simulink model "eovsa_corr_300mhz"  (R2012b)
settings: Solver=VariableStepDiscrete  SolverMode=SingleTasking  StartTime=0.0  StopTime=5000  RelTol=1e-3
undefined symbols (not defined in the file or in its folder): A, B, gcbh, PCIN, sfp, xlBlockLoadCallback, xlipgetpartsetting
libraries: xbsIndex_r4 x5996, casper_library_misc x52, simulink x33, dspsigops x24, xps_library x15, casper_library_delays x2
(part 3 of 65)

== system eovsa_corr_300mhz/FPGA_pps ==
  Slice29 : xbsIndex_r4/Slice  nbits=1  boolean_output=on  mode=Upper Bit Location + Width  bit1=0  base1=MSB of Input  bit0=0  base0=LSB of Input  dbl_ovrd=off  block_type=slice
  count_1sec : xbsIndex_r4/Counter  cnt_type=Count Limited  cnt_to=( fpga_clk * ( 10 ^ 6 ) ) - 1  operation=Up  start_count=0  cnt_by_val=1  arith_type=Unsigned  n_bits=ceil( log2( fpga_clk * ( 10 ^ 6 ) ) )  bin_pt=0  load_pin=off  rst=off  en=off  explicit_period=on  period=1  dbl_ovrd=off  use_behavioral_HDL=off  implementation=DSP48  block_type=counter
      settings: block_version=11.4
  edge_detect6 : Subsystem  AncestorBlock=casper_library_misc/edge_detect  mask(edge_detect){edge=Falling, polarity=Active High, x_in=[0 0.08 0.08 0.16 0.16 0.24 0.24 0.32 0.32 0.4], y_in=[1  1 -1 -1 -1 -1 -1 -1 -1 -1], x_out=[0.6 0.68 0.68 0.76 0.76 0.84 0.84 0.92 0.92 1], y_out=[-1 -1  1  1 -1 -1 -1 -1 -1 -1]}
      mask prompts: edge "Edge Type"; polarity "Output Polarity"; x_in "Input X Positions"; y_in "Input Y Positions"; x_out "Output X Positions"; y_out "Output Y Positions"
      mask help: Output is active for one-cycle after each edge of the specified type (i.e. rising, falling or both).
      mask init: same as eovsa_corr_300mhz/edge_detect1
      settings: AttributesFormatString=|
      | falling edges
      | active high
      mask Help: Output is active for one-cycle after each edge of the specified type (i.e. rising, falling, or both).  Latency is zero.
      mask TypeOptions edge: Rising | Falling | Both
      mask TypeOptions polarity: Active High | Active Low
      mask Display:
      | plot(x_in_num,0.5+y_in_num*0.2);
      | plot(x_out_num,0.5+y_out_num*0.2);
  pps : Outport
  wires:
  count_1sec/1 -> Slice29/1
  Slice29/1 -> edge_detect6/1(in)
  edge_detect6/1(out) -> pps/1

== system eovsa_corr_300mhz/Subsystem ==
  In1 : Inport
  Delay{16..23,28..30,32,34,37} (14 alike) : xbsIndex_r4/Delay  rst=off  infoeditControl=Selection of Reset will increase slice count due to use of real FFs and instead of SRLs  en=off  latency=1  dbl_ovrd=off  reg_retiming=off  block_type=delay
      settings: block_version=11.4
  Out1 : Outport
  Out2 : Outport  Port=2
  Out3 : Outport  Port=3
  Out4 : Outport  Port=4
  Out5 : Outport  Port=5
  Out6 : Outport  Port=6
  Out7 : Outport  Port=7
  Out8 : Outport  Port=8
  wires:
  Delay21/1 -> Delay37/1, Delay34/1
  Delay19/1 -> Delay28/1, Delay29/1
  Delay29/1 -> Out4/1
  Delay32/1 -> Out6/1
  Delay30/1 -> Out5/1
  In1/1 -> Delay16/1, Delay17/1
  Delay18/1 -> Delay22/1, Delay23/1
  Delay20/1 -> Delay32/1, Delay30/1
  Delay22/1 -> Out1/1
  Delay34/1 -> Out7/1
  Delay23/1 -> Out2/1
  Delay16/1 -> Delay19/1, Delay18/1
  Delay28/1 -> Out3/1
  Delay17/1 -> Delay21/1, Delay20/1
  Delay37/1 -> Out8/1

== system eovsa_corr_300mhz/acc_sync ==
  note: Count number of ADC overflows in an accumulation.
  sync : Inport
  acc_len : Inport  Port=2
  acc_start_skip : Inport  Port=3
  adc_over : Inport  Port=4
  AddSub : xbsIndex_r4/AddSub  mode=Addition  use_carryin=off  use_carryout=off  en=off  latency=1  precision=User Defined  arith_type=Unsigned  n_bits=16  bin_pt=0  quantization=Truncate  overflow=Wrap  dbl_ovrd=off  use_behavioral_HDL=off  hw_selection=DSP48  pipelined=off  block_type=addsub
  Count_FFT_frames1 : xbsIndex_r4/Counter  cnt_type=Free Running  cnt_to=0  operation=Up  start_count=0  cnt_by_val=1  arith_type=Unsigned  n_bits=32  bin_pt=0  load_pin=off  rst=on  en=on  explicit_period=off  period=1  dbl_ovrd=off  use_behavioral_HDL=off  implementation=DSP48  use_rpm=off  block_type=counter
  Delay{1,3..6,8..11} (9 alike) : xbsIndex_r4/Delay  rst=off  infoeditControl=Selection of Reset will increase slice count due to use of real FFs and instead of SRLs  en=off  latency=1  dbl_ovrd=off  reg_retiming=off  block_type=delay
      settings: block_version=11.4
  Delay2 : xbsIndex_r4/Delay  rst=off  infoeditControl=Selection of Reset will increase slice count due to use of real FFs and instead of SRLs  en=off  latency=2  dbl_ovrd=off  reg_retiming=on  block_type=delay
      settings: block_version=11.4
  Delay7 : xbsIndex_r4/Delay  rst=off  infoeditControl=Selection of Reset will increase slice count due to use of real FFs and instead of SRLs  en=off  latency=2  dbl_ovrd=off  reg_retiming=off  block_type=delay
      settings: block_version=11.4
  Register1 : xbsIndex_r4/Register  init=0  rst=off  en=on  dbl_ovrd=off  block_type=register
      settings: block_version=11.4
  Relational2 : xbsIndex_r4/Relational  mode=a=b  en=off  latency=1  dbl_ovrd=off  block_type=relational
  Relational3 : xbsIndex_r4/Relational  mode=a=b  en=off  latency=1  dbl_ovrd=off  block_type=relational
  adc_overflow_count : xbsIndex_r4/Counter  cnt_type=Free Running  cnt_to=5  operation=Up  start_count=0  cnt_by_val=1  arith_type=Unsigned  n_bits=32  bin_pt=0  load_pin=off  rst=on  en=on  explicit_period=off  period=1  dbl_ovrd=off  use_behavioral_HDL=off  implementation=DSP48  use_rpm=off  block_type=counter
  edge_detect : Subsystem  AncestorBlock=casper_library_misc/edge_detect  mask(edge_detect){edge=Rising, polarity=Active High, x_in=[0 0.08 0.08 0.16 0.16 0.24 0.24 0.32 0.32 0.4], y_in=[-1 -1  1  1  1  1  1  1  1  1], x_out=[0.6 0.68 0.68 0.76 0.76 0.84 0.84 0.92 0.92 1], y_out=[-1 -1  1  1 -1 -1 -1 -1 -1 -1]}
      mask prompts: edge "Edge Type"; polarity "Output Polarity"; x_in "Input X Positions"; y_in "Input Y Positions"; x_out "Output X Positions"; y_out "Output Y Positions"
      mask help: Output is active for one-cycle after each edge of the specified type (i.e. rising, falling or both).
      mask init: same as eovsa_corr_300mhz/edge_detect1
      settings: AttributesFormatString=|
      | rising edges
      | active high
      mask Help: Output is active for one-cycle after each edge of the specified type (i.e. rising, falling, or both).  Latency is zero.
      mask TypeOptions edge: Rising | Falling | Both
      mask TypeOptions polarity: Active High | Active Low
      mask Display:
      | plot(x_in_num,0.5+y_in_num*0.2);
      | plot(x_out_num,0.5+y_out_num*0.2);
  edge_detect1 : Subsystem  AncestorBlock=casper_library_misc/edge_detect  mask(edge_detect){edge=Rising, polarity=Active High, x_in=[0 0.08 0.08 0.16 0.16 0.24 0.24 0.32 0.32 0.4], y_in=[-1 -1  1  1  1  1  1  1  1  1], x_out=[0.6 0.68 0.68 0.76 0.76 0.84 0.84 0.92 0.92 1], y_out=[-1 -1  1  1 -1 -1 -1 -1 -1 -1]}
      mask prompts: edge "Edge Type"; polarity "Output Polarity"; x_in "Input X Positions"; y_in "Input Y Positions"; x_out "Output X Positions"; y_out "Output Y Positions"
      mask help: Output is active for one-cycle after each edge of the specified type (i.e. rising, falling or both).
      mask init: same as eovsa_corr_300mhz/edge_detect1
      settings: AttributesFormatString=|
      | rising edges
      | active high
      mask Help: Output is active for one-cycle after each edge of the specified type (i.e. rising, falling, or both).  Latency is zero.
      mask TypeOptions edge: Rising | Falling | Both
      mask TypeOptions polarity: Active High | Active Low
      mask Display:
      | plot(x_in_num,0.5+y_in_num*0.2);
      | plot(x_out_num,0.5+y_out_num*0.2);
  gen_N_pps : Subsystem  mask{fpga_clk_sub=fpga_clk, n_pps_sub=n_pps}
      mask prompts: fpga_clk_sub "FPGA Clock Frequency (MHz)"; n_pps_sub "Number of pulses per second (> 1)"
      mask init:
      | count_pulses = ceil(fpga_clk_sub * (10 ^ 6) / n_pps_sub);
  pulse generator : Subsystem  mask{period=2 ^ ( freq_chan - 1 )}
      mask prompts: period "Period (clock cycles)"
  acc_end : Outport
  adc_overflow : Outport  Port=2
  wires:
  adc_over/1 -> Delay7/1
  sync/1 -> pulse generator/1(sync), gen_N_pps/1(sync)
  pulse generator/1(pulse) -> Delay2/1
  Count_FFT_frames1/1 -> Delay3/1, Delay5/1
  acc_start_skip/1 -> Delay4/1, AddSub/2
  Relational2/1 -> edge_detect/1(in)
  edge_detect/1(out) -> Delay9/1
  Relational3/1 -> edge_detect1/1(in)
  edge_detect1/1(out) -> Delay10/1
  acc_len/1 -> AddSub/1
  AddSub/1 -> Delay6/1
  adc_overflow_count/1 -> Register1/1
  Register1/1 -> adc_overflow/1
  gen_N_pps/1(n_pps) -> Delay8/1
  Delay1/1 -> acc_end/1
  Delay2/1 -> Count_FFT_frames1/2
  Delay3/1 -> Relational2/1
  Delay4/1 -> Relational2/2
  Delay5/1 -> Relational3/1
  Delay6/1 -> Relational3/2
  Delay7/1 -> Delay11/1
  Delay8/1 -> Count_FFT_frames1/1
  Delay9/1 -> adc_overflow_count/1
  Delay10/1 -> Delay1/1, Register1/2
  Delay11/1 -> adc_overflow_count/2

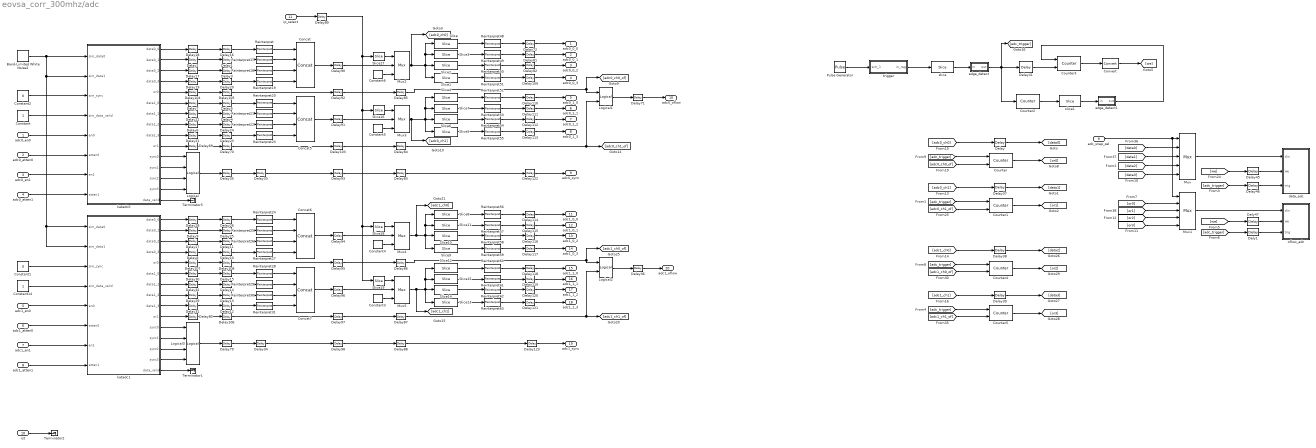
== system eovsa_corr_300mhz/adc ==
  adc0_en0 : Inport
  adc0_atten0 : Inport  Port=2
  adc0_en1 : Inport  Port=3
  adc0_atten1 : Inport  Port=4
  adc1_en0 : Inport  Port=5
  adc1_atten0 : Inport  Port=6
  adc1_en1 : Inport  Port=7
  adc1_atten1 : Inport  Port=8
  adc_snap_sel : Inport  Port=9
  rst : Inport  Port=10
  ip_select : Inport  Port=11
  Band-Limited White Noise2 : simulink/Sources/Band-Limited White Noise  Cov=[0.5]  Ts=1  seed=[23341]
  Concat{,5..7} (4 alike) : xbsIndex_r4/Concat  num_inputs=4  dbl_ovrd=off  block_type=concat
  Constant : Constant  SampleTime=1/4
  Constant1 : Constant  Value=0  SampleTime=1/4
  Constant14 : Constant  SampleTime=1/4
  Constant2 : Constant  Value=0  SampleTime=1/4
  Constant{3..6} (4 alike) : xbsIndex_r4/Constant  const=0  gui_display_data_type=Fixed-point  arith_type=Unsigned  n_bits=32  bin_pt=0  preci_type=Single  exp_width=8  frac_width=24  explicit_period=on  period=1  equ=P=C  opselect=C  inp2=PCIN>>17  opr=+  inp1=P  carry=CIN  dbl_ovrd=off  block_type=constant
      settings: block_version=11.4
  Convert : xbsIndex_r4/Convert  gui_display_data_type=Fixed-point  arith_type=Boolean  n_bits=16  bin_pt=14  float_type=Single  exp_bits=8  fraction_bits=24  quantization=Truncate  overflow=Wrap  en=off  latency=0  dbl_ovrd=off  pipeline=off  block_type=convert
      settings: block_version=11.4
  Counter{,1,4..5} (4 alike) : xbsIndex_r4/Counter  cnt_type=Free Running  cnt_to=Inf  operation=Up  start_count=0  cnt_by_val=1  arith_type=Unsigned  n_bits=16  bin_pt=0  load_pin=off  rst=on  en=on  explicit_period=off  period=1  dbl_ovrd=off  use_behavioral_HDL=off  implementation=Fabric  block_type=counter
      settings: block_version=11.4
  Counter2 : xbsIndex_r4/Counter  cnt_type=Free Running  cnt_to=Inf  operation=Up  start_count=0  cnt_by_val=1  arith_type=Unsigned  n_bits=4  bin_pt=0  load_pin=off  rst=on  en=off  explicit_period=on  period=1  dbl_ovrd=off  use_behavioral_HDL=off  implementation=Fabric  block_type=counter
      settings: block_version=11.4
  Counter3 : xbsIndex_r4/Counter  cnt_type=Free Running  cnt_to=Inf  operation=Up  start_count=0  cnt_by_val=1  arith_type=Unsigned  n_bits=1  bin_pt=0  load_pin=off  rst=on  en=on  explicit_period=off  period=1  dbl_ovrd=off  use_behavioral_HDL=off  implementation=Fabric  block_type=counter
      settings: block_version=11.4
  Delay{,2,6..9,17..19,21..22,27..32,35..39,41,45..46,69,71..72,79..98,103..104,107,109..123} (66 alike) : xbsIndex_r4/Delay  rst=off  infoeditControl=Selection of Reset will increase slice count due to use of real FFs and instead of SRLs  en=off  latency=1  dbl_ovrd=off  reg_retiming=on  block_type=delay
      Delay settings: block_version=11.4
      Delay37 settings: block_version=11.4
      Delay38 settings: block_version=11.4
      Delay39 settings: block_version=11.4
      Delay41 settings: block_version=11.4
      Delay45 settings: block_version=11.4
      Delay46 settings: block_version=11.4
  Delay{1,3..5,10..16,20,23..26,33..34,70,105..106,108} (22 alike) : xbsIndex_r4/Delay  rst=off  infoeditControl=Selection of Reset will increase slice count due to use of real FFs and instead of SRLs  en=off  latency=delay - 1  dbl_ovrd=off  reg_retiming=on  block_type=delay
  Dely1 : xbsIndex_r4/Delay  rst=off  infoeditControl=Selection of Reset will increase slice count due to use of real FFs and instead of SRLs  en=off  latency=1  dbl_ovrd=off  reg_retiming=on  block_type=delay
      settings: block_version=11.4
  Dely47 : xbsIndex_r4/Delay  rst=off  infoeditControl=Selection of Reset will increase slice count due to use of real FFs and instead of SRLs  en=off  latency=1  dbl_ovrd=off  reg_retiming=on  block_type=delay
      settings: block_version=11.4
  Logical : xbsIndex_r4/Logical  logical_function=OR  inputs=4  en=off  latency=0  precision=Full  arith_type=Unsigned  n_bits=16  bin_pt=0  align_bp=on  dbl_ovrd=off  block_type=logical
  Logical1 : xbsIndex_r4/Logical  logical_function=OR  inputs=2  en=off  latency=0  precision=Full  arith_type=Unsigned  n_bits=16  bin_pt=0  align_bp=on  dbl_ovrd=off  block_type=logical
  Logical2 : xbsIndex_r4/Logical  logical_function=OR  inputs=2  en=off  latency=0  precision=Full  arith_type=Unsigned  n_bits=16  bin_pt=0  align_bp=on  dbl_ovrd=off  block_type=logical
  Logical3 : xbsIndex_r4/Logical  logical_function=OR  inputs=4  en=off  latency=0  precision=Full  arith_type=Unsigned  n_bits=16  bin_pt=0  align_bp=on  dbl_ovrd=off  block_type=logical
  Mux : xbsIndex_r4/Mux  inputs=4  en=off  latency=1  precision=Full  arith_type=Unsigned  n_bits=16  bin_pt=14  quantization=Truncate  overflow=Wrap  dbl_ovrd=off  block_type=mux
      settings: block_version=11.4
  Mux1 : xbsIndex_r4/Mux  inputs=4  en=off  latency=1  precision=Full  arith_type=Unsigned  n_bits=16  bin_pt=14  quantization=Truncate  overflow=Wrap  dbl_ovrd=off  block_type=mux
      settings: block_version=11.4
  Mux{2..5} (4 alike) : xbsIndex_r4/Mux  inputs=2  en=off  latency=1  precision=Full  arith_type=Unsigned  n_bits=16  bin_pt=14  quantization=Truncate  overflow=Wrap  dbl_ovrd=off  block_type=mux
      settings: block_version=11.4
  Pulse Generator : DiscretePulseGenerator  Period=50  PulseWidth=5  PhaseDelay=5
  Reinterpret{,17..31} (16 alike) : xbsIndex_r4/Reinterpret  force_arith_type=on  arith_type=Unsigned  force_bin_pt=on  bin_pt=0  block_type=reinterpret
      settings: infoedit="Changes signal type without altering the binary representation.   You can changed the signal between signed and unsigned, and relocate the binary point.<br><br>Hardware notes: In hardware this block costs nothing.<br><br>Example:  Suppose the input is 6 bits wide, signed, with 2 fractional bits, and the output is forced to unsigned with 0 fractional bits.  Then an input of -2.0 (1110.00 in binary 2's complement) becomes an output of 56 (111000 in binary)."
  Reinterpret{48..63} (16 alike) : xbsIndex_r4/Reinterpret  force_arith_type=on  arith_type="Signed  (2's comp)"  force_bin_pt=on  bin_pt=7  block_type=reinterpret
      settings: infoedit="Changes signal type without altering the binary representation.   You can changed the signal between signed and unsigned, and relocate the binary point.<br><br>Hardware notes: In hardware this block costs nothing.<br><br>Example:  Suppose the input is 6 bits wide, signed, with 2 fractional bits, and the output is forced to unsigned with 0 fractional bits.  Then an input of -2.0 (1110.00 in binary 2's complement) becomes an output of 56 (111000 in binary)."
  Slice{,4,8,12} (4 alike) : xbsIndex_r4/Slice  nbits=8  boolean_output=off  mode=Upper Bit Location + Width  bit1=0  base1=MSB of Input  bit0=0  base0=LSB of Input  dbl_ovrd=off  block_type=slice
  Slice{1,5,9,13} (4 alike) : xbsIndex_r4/Slice  nbits=8  boolean_output=off  mode=Lower Bit Location + Width  bit1=0  base1=MSB of Input  bit0=0  base0=LSB of Input  dbl_ovrd=off  block_type=slice
  Slice{2,6,10,14} (4 alike) : xbsIndex_r4/Slice  nbits=8  boolean_output=off  mode=Lower Bit Location + Width  bit1=0  base1=MSB of Input  bit0=8  base0=LSB of Input  dbl_ovrd=off  block_type=slice
  Slice{3,7,11,15} (4 alike) : xbsIndex_r4/Slice  nbits=8  boolean_output=off  mode=Lower Bit Location + Width  bit1=0  base1=MSB of Input  bit0=16  base0=LSB of Input  dbl_ovrd=off  block_type=slice
  Slice16 : xbsIndex_r4/Slice  nbits=1  boolean_output=off  mode=Lower Bit Location + Width  bit1=0  base1=MSB of Input  bit0=1  base0=LSB of Input  dbl_ovrd=off  block_type=slice
  Slice17 : xbsIndex_r4/Slice  nbits=1  boolean_output=off  mode=Lower Bit Location + Width  bit1=0  base1=MSB of Input  bit0=0  base0=LSB of Input  dbl_ovrd=off  block_type=slice
  Slice18 : xbsIndex_r4/Slice  nbits=1  boolean_output=off  mode=Lower Bit Location + Width  bit1=0  base1=MSB of Input  bit0=2  base0=LSB of Input  dbl_ovrd=off  block_type=slice
  Slice19 : xbsIndex_r4/Slice  nbits=1  boolean_output=off  mode=Lower Bit Location + Width  bit1=0  base1=MSB of Input  bit0=3  base0=LSB of Input  dbl_ovrd=off  block_type=slice
  Terminator1 : Terminator
  Terminator2 : Terminator
  Terminator5 : Terminator
  data_adc : Subsystem  Tag=casper:snapshot  AncestorBlock=casper_library_scopes/snapshot  mask(snapshot){storage=bram, dram_dimm=1, dram_clock=200, nsamples=11, data_width=32, offset=off, circap=off, value=off, use_dsp48=on}
      mask prompts: storage "Storage medium"; dram_dimm "DRAM dimm"; dram_clock "DRAM clock rate"; nsamples "Number of Samples (2^?)"; data_width "Data width"; offset "Start delay support"; circap "Circular capture support"; value "Extra value capture support"; use_dsp48 "Use DSP48s to implement counters"
      mask help:
      | Standard snap block, but with the following optional extras;
      |  1) Optionally delay the fabric trigger by a user-specified number of valids.
      |  2) Capture continuously after a trigger until a stop pulse is received. Data is captured into BRAM continuously, with old data being overwritten until a stop command is received. Then stop capturing when memory is filled. This enables you to get some data before and some data after the stop pulse. Use the 'tr_en_cnt' register to determine where you are in your vector. 'Addr' register's MSb now indicates 'busy capturing'.
      |  3) Optionally capture a value on an input port to a register at the same time as the first data sample.
      |  4) Implement counters using DSP48Es to save resources.
      mask init: same as eovsa_corr_300mhz/rx_hdr
      mask TypeOptions storage: bram | dram
      mask Callback storage: snapshot_callback();
      mask TypeOptions dram_dimm: 1 | 2 | 3 | 4
      mask TypeOptions dram_clock: 200 | 250 | 266 | 300 | 333
      mask TypeOptions data_width: 8 | 16 | 32 | 64 | 128
  edge_detect : Subsystem  AncestorBlock=casper_library_misc/edge_detect  mask(edge_detect){edge=Rising, polarity=Active High, x_in=[0 0.08 0.08 0.16 0.16 0.24 0.24 0.32 0.32 0.4], y_in=[-1 -1  1  1  1  1  1  1  1  1], x_out=[0.6 0.68 0.68 0.76 0.76 0.84 0.84 0.92 0.92 1], y_out=[-1 -1  1  1 -1 -1 -1 -1 -1 -1]}
      mask prompts: edge "Edge Type"; polarity "Output Polarity"; x_in "Input X Positions"; y_in "Input Y Positions"; x_out "Output X Positions"; y_out "Output Y Positions"
      mask help: Output is active for one-cycle after each edge of the specified type (i.e. rising, falling or both).
      mask init: same as eovsa_corr_300mhz/edge_detect1
      settings: AttributesFormatString=|
      | rising edges
      | active high
      mask Help: Output is active for one-cycle after each edge of the specified type (i.e. rising, falling, or both).  Latency is zero.
      mask TypeOptions edge: Rising | Falling | Both
      mask TypeOptions polarity: Active High | Active Low
      mask Display:
      | plot(x_in_num,0.5+y_in_num*0.2);
      | plot(x_out_num,0.5+y_out_num*0.2);
  edge_detect1 : Subsystem  AncestorBlock=casper_library_misc/edge_detect  mask(edge_detect){edge=Falling, polarity=Active High, x_in=[0 0.08 0.08 0.16 0.16 0.24 0.24 0.32 0.32 0.4], y_in=[1  1 -1 -1 -1 -1 -1 -1 -1 -1], x_out=[0.6 0.68 0.68 0.76 0.76 0.84 0.84 0.92 0.92 1], y_out=[-1 -1  1  1 -1 -1 -1 -1 -1 -1]}
      mask prompts: edge "Edge Type"; polarity "Output Polarity"; x_in "Input X Positions"; y_in "Input Y Positions"; x_out "Output X Positions"; y_out "Output Y Positions"
      mask help: Output is active for one-cycle after each edge of the specified type (i.e. rising, falling or both).
      mask init: same as eovsa_corr_300mhz/edge_detect1
      settings: AttributesFormatString=|
      | falling edges
      | active high
      mask Help: Output is active for one-cycle after each edge of the specified type (i.e. rising, falling, or both).  Latency is zero.
      mask TypeOptions edge: Rising | Falling | Both
      mask TypeOptions polarity: Active High | Active Low
      mask Display:
      | plot(x_in_num,0.5+y_in_num*0.2);
      | plot(x_out_num,0.5+y_out_num*0.2);
  katadc0 : Subsystem  Tag=xps:katadc  AncestorBlock=xps_library/katadc  mask(katadc){adc_brd=adc0, adc_interleave=off, bypass_auto=off, en_gain=on, adc_clk_rate=1200, sample_period=1}
      mask prompts: adc_brd "ADC board"; adc_interleave "ADC interleave mode"; bypass_auto "Bypass auto config"; en_gain "Enable gain"; adc_clk_rate "ADC sampling rate (MHz)"; sample_period "Sample period"
      mask init:
      | name = gcb;
      | katadc_init(gcb, ...
      |     'name', name, ...
      |     'adc_brd', adc_brd, ...
      |     'adc_interleave', adc_interleave, ...
      |     'bypass_auto', bypass_auto, ...
      |     'en_gain', en_gain, ...
      |     'adc_clk_rate', adc_clk_rate, ...
      |     'sample_period', sample_period);
      mask TypeOptions adc_brd: adc0 | adc1
  katadc1 : Subsystem  Tag=xps:katadc  AncestorBlock=xps_library/katadc  mask(katadc){adc_brd=adc1, adc_interleave=off, bypass_auto=off, en_gain=on, adc_clk_rate=1200, sample_period=1}
      mask prompts: adc_brd "ADC board"; adc_interleave "ADC interleave mode"; bypass_auto "Bypass auto config"; en_gain "Enable gain"; adc_clk_rate "ADC sampling rate (MHz)"; sample_period "Sample period"
      mask init: same as eovsa_corr_300mhz/adc/katadc0
      mask TypeOptions adc_brd: adc0 | adc1
  oflow_adc : Subsystem  Tag=casper:snapshot  AncestorBlock=casper_library_scopes/snapshot  mask(snapshot){storage=bram, dram_dimm=1, dram_clock=200, nsamples=11, data_width=16, offset=off, circap=off, value=off, use_dsp48=on}
      mask prompts: storage "Storage medium"; dram_dimm "DRAM dimm"; dram_clock "DRAM clock rate"; nsamples "Number of Samples (2^?)"; data_width "Data width"; offset "Start delay support"; circap "Circular capture support"; value "Extra value capture support"; use_dsp48 "Use DSP48s to implement counters"
      mask help:
      | Standard snap block, but with the following optional extras;
      |  1) Optionally delay the fabric trigger by a user-specified number of valids.
      |  2) Capture continuously after a trigger until a stop pulse is received. Data is captured into BRAM continuously, with old data being overwritten until a stop command is received. Then stop capturing when memory is filled. This enables you to get some data before and some data after the stop pulse. Use the 'tr_en_cnt' register to determine where you are in your vector. 'Addr' register's MSb now indicates 'busy capturing'.
      |  3) Optionally capture a value on an input port to a register at the same time as the first data sample.
      |  4) Implement counters using DSP48Es to save resources.
      mask init: same as eovsa_corr_300mhz/rx_hdr
      mask TypeOptions storage: bram | dram
      mask Callback storage: snapshot_callback();
      mask TypeOptions dram_dimm: 1 | 2 | 3 | 4
      mask TypeOptions dram_clock: 200 | 250 | 266 | 300 | 333
      mask TypeOptions data_width: 8 | 16 | 32 | 64 | 128
  slice : xbsIndex_r4/Slice  nbits=1  boolean_output=on  mode=Lower Bit Location + Width  bit1=0  base1=MSB of Input  bit0=0  base0=LSB of Input  dbl_ovrd=off  block_type=slice
  slice1 : xbsIndex_r4/Slice  nbits=1  boolean_output=on  mode=Upper Bit Location + Width  bit1=0  base1=MSB of Input  bit0=0  base0=LSB of Input  dbl_ovrd=off  block_type=slice
  trigger : Subsystem  Tag=xps:sw_reg  AncestorBlock=xps_library/software_register  mask(swreg){mode=one value, io_dir=From Processor, io_delay=0, sample_period=1, names=reg, bitwidths=32, arith_types=0, bin_pts=0, sim_port=on, show_format=off}
      mask prompts: io_dir "I/O direction"; io_delay "I/O delay"; sample_period "Sample period"; names "Name:"; bitwidths "Bitwidth:"; arith_types "Type (ufix=0, fix=1, bool=2):"; bin_pts "Binary pt:"; sim_port "Provide sim input/output?"; show_format "Print format string?"
      mask init:
      | swreg_init(gcb)
      settings: AttributesFormatString=1input
      mask TypeOptions mode: one value | fields of equal size | fields of arbitrary size
      mask Callback mode: swreg_cb(gcb);
      mask TypeOptions io_dir: To Processor | From Processor
      mask Callback io_dir:
      | mask_enables = get_param(gcb, 'MaskEnables');
      | mask_names = get_param(gcb, 'MaskNames');
      | if strcmp(get_param(gcb, 'io_dir'), 'To Processor'),
      |     mask_enables{ismember(mask_names, 'sample_period')} = 'off';
      | else
      |     mask_enables{ismember(mask_names, 'sample_period')} = 'on';
      | end
      | set_param(gcb, 'MaskEnables', mask_enables);
      mask Callback bitwidths:
      | swreg_maskcheck(gcb);
      | % blk = gcb;
      | % mode = get_param(blk, 'mode');
      | % current_widths = eval(get_param(blk, 'bitwidths'));
      | % if (strcmp(mode, 'one value') || strcmp(mode, 'fields of equal size')) && (length(current_widths) > 1),
      | %     error('Only one width may be specified for this mode.');
      | % elseif strcmp(mode, 'fields of arbitrary size')
      | %     current_names = textscan(strtrim(strrep(strrep(get_param(blk, 'names'), ']', ''), '[', '')), '%s');
      | %     current_names = current_names{1};
      | %     numios = length(current_names);
      | %     if length(current_widths) ~= numios,
      | %         error('%d field names specified, but %d widths?', numios, length(current_widths));
      | %     end
      | % end
      | % total_width = 0;
      | % for ctr = 1 : length(current_widths),
      | %     total_width = total_width + current_widths(ctr);
      | % end
      | % if total_width > 32,
      | %     error('Total width must be 32 or less, set to %d.', total_width);
      | % end
      mask Callback arith_types:
      | [numios, ~, ~, ~, current_types] = swreg_maskcheck(gcb);
      | % blk = gcb;
      | % mode = get_param(blk, 'mode');
      | % current_types = eval(get_param(blk, 'arith_types'));
      | % numios = length(current_types);
      | % if (strcmp(mode, 'one value') || strcmp(mode, 'fields of equal size')) && (length(current_types) > 1),
      | %     error('Only one type may be specified for this mode.');
      | % elseif strcmp(mode, 'fields of arbitrary size')
      | %     current_names = textscan(strtrim(strrep(strrep(get_param(blk, 'names'), ']', ''), '[', '')), '%s');
      | %     current_names = current_names{1};
      | %     numios = length(current_names);
      | %     if length(current_types) ~= numios,
      | %         error('%d field names specified, but %d types?', numios, length(current_types));
      | %     end
      | % end
      | problem = 0;
      | for ctr = 1 : numios,
      |     t = current_types(ctr);
      |     if (t < 0) || (t > 2),
      |         problem = t;
      |         ctr = numios + 1;
      |     end
      | end
      | if problem ~= 0,
      |     error('Type cannot be %i, must be 0, 1 or 2.', problem);
      | end
      mask Callback bin_pts:
      | swreg_maskcheck(gcb);
      | % blk = gcb;
      | % mode = get_param(blk, 'mode');
      | % current_bins = eval(get_param(blk, 'bin_pts'));
      | % if (strcmp(mode, 'one value') || strcmp(mode, 'fields of equal size')) && (length(current_bins) > 1),
      | %     error('Only one binary pt may be specified for this mode.');
      | % elseif strcmp(mode, 'fields of arbitrary size')
      | %     current_names = textscan(strtrim(strrep(strrep(get_param(blk, 'names'), ']', ''), '[', '')), '%s');
      | %     current_names = current_names{1};
      | %     numios = length(current_names);
      | %     if length(current_bins) ~= numios,
      | %         error('%d field names specified, but %d binary pts?', numios, length(current_bins));
      | %     end
      | % end
  adc0_0_0 : Outport
  adc0_0_1 : Outport  Port=2
  adc0_0_2 : Outport  Port=3
  adc0_0_3 : Outport  Port=4
  adc0_1_0 : Outport  Port=5
  adc0_1_1 : Outport  Port=6
  adc0_1_2 : Outport  Port=7
  adc0_1_3 : Outport  Port=8
  adc0_sync : Outport  Port=9
  adc0_oflow : Outport  Port=10
  adc1_0_0 : Outport  Port=11
  adc1_0_1 : Outport  Port=12
  adc1_0_2 : Outport  Port=13
  adc1_0_3 : Outport  Port=14
  adc1_1_0 : Outport  Port=15
  adc1_1_1 : Outport  Port=16
  adc1_1_2 : Outport  Port=17
  adc1_1_3 : Outport  Port=18
  adc1_sync : Outport  Port=19
  adc1_oflow : Outport  Port=20
  wires:
  katadc0/1(data0_0) -> Delay18/1
  katadc0/2(data0_1) -> Delay2/1
  katadc0/3(data0_2) -> Delay17/1
  katadc0/4(data0_3) -> Delay19/1
  Delay18/1 -> Delay16/1
  katadc1/2(data0_1) -> Delay9/1
  katadc1/3(data0_2) -> Delay27/1
  katadc1/4(data0_3) -> Delay8/1
  Logical/1 -> Delay35/1
  katadc0/11(sync0) -> Logical/1
  katadc0/12(sync1) -> Logical/2
  katadc0/13(sync2) -> Logical/3
  katadc0/14(sync3) -> Logical/4
  katadc0/15(data_valid) -> Terminator5/1
  katadc0/6(data1_0) -> Delay7/1
  katadc0/7(data1_1) -> Delay22/1
  katadc0/8(data1_2) -> Delay6/1
  katadc0/9(data1_3) -> Delay21/1
  katadc1/1(data0_0) -> Delay28/1
  katadc1/7(data1_1) -> Delay32/1
  katadc1/8(data1_2) -> Delay29/1
  katadc1/9(data1_3) -> Delay31/1
  katadc1/6(data1_0) -> Delay30/1
  katadc1/11(sync0) -> Logical3/1
  katadc1/12(sync1) -> Logical3/2
  katadc1/13(sync2) -> Logical3/3
  katadc1/14(sync3) -> Logical3/4
  katadc1/15(data_valid) -> Terminator1/1
  Logical3/1 -> Delay79/1
  Logical2/1 -> Delay36/1
  Constant1/1 -> katadc1/3(sim_sync)
  Constant14/1 -> katadc1/4(sim_data_valid)
  adc1_en1/1 -> katadc1/7(en1)
  adc1_atten1/1 -> katadc1/8(atten1)
  Band-Limited White Noise2/1 -> katadc0/1(sim_data0), katadc0/2(sim_data1), katadc1/1(sim_data0), katadc1/2(sim_data1)
  Constant2/1 -> katadc0/3(sim_sync)
  Constant/1 -> katadc0/4(sim_data_valid)
  adc0_en0/1 -> katadc0/5(en0)
  adc0_atten0/1 -> katadc0/6(atten0)
  adc0_en1/1 -> katadc0/7(en1)
  adc0_atten1/1 -> katadc0/8(atten1)
  adc1_en0/1 -> katadc1/5(en0)
  adc1_atten0/1 -> katadc1/6(atten0)
  Delay2/1 -> Delay1/1
  Delay17/1 -> Delay3/1
  Delay19/1 -> Delay20/1
  Delay7/1 -> Delay5/1
  Delay22/1 -> Delay4/1
  Delay6/1 -> Delay24/1
  Delay21/1 -> Delay23/1
  Delay28/1 -> Delay26/1
  Delay9/1 -> Delay25/1
  Delay27/1 -> Delay11/1
  Delay8/1 -> Delay10/1
  Delay30/1 -> Delay15/1
  Delay32/1 -> Delay14/1
  Delay29/1 -> Delay13/1
  Delay31/1 -> Delay12/1
  Delay33/1 -> Delay93/1
  Delay34/1 -> Delay98/1
  Delay36/1 -> adc1_oflow/1
  Mux/1 -> data_adc/1(din)
  [adc0_ch0] -> Delay/1
  [adc0_ch1] -> Delay37/1
  [adc0_ch0_of] -> Counter/2
  [adc0_ch1_of] -> Counter1/2
  [adc_trigger] -> Counter/1
  [adc_trigger] -> Counter1/1
  Pulse Generator/1 -> trigger/1(sim_1)
  trigger/1(in_reg) -> slice/1
  slice/1 -> edge_detect/1(in)
  slice1/1 -> edge_detect1/1(in)
  Counter2/1 -> slice1/1
  edge_detect1/1(out) -> Counter3/1
  Counter3/1 -> Convert/1
  Convert/1 -> [we]
  Delay41/1 -> Counter3/2
  edge_detect/1(out) -> Delay41/1, [adc_trigger], Counter2/1
  [adc1_ch0] -> Delay38/1
  [adc1_ch1] -> Delay39/1
  [adc_trigger] -> Counter4/1
  [adc_trigger] -> Counter5/1
  [adc1_ch1_of] -> Counter5/2
  [adc1_ch0_of] -> Counter4/2
  adc_snap_sel/1 -> Mux/1, Mux1/1
  [data0] -> Mux/2
  [data1] -> Mux/3
  Delay/1 -> [data0]
  Counter/1 -> [or0]
  Delay37/1 -> [data1]
  Counter1/1 -> [or1]
  Delay38/1 -> [data2]
  Counter4/1 -> [or2]
  Delay39/1 -> [data3]
  Counter5/1 -> [or3]
  [or0] -> Mux1/2
  [or1] -> Mux1/3
  [data2] -> Mux/4
  [data3] -> Mux/5
  [or2] -> Mux1/4
  [or3] -> Mux1/5
  [we] -> Delay45/1
  [adc_trigger] -> Delay46/1
  [we] -> Dely47/1
  [adc_trigger] -> Dely1/1
  Delay45/1 -> data_adc/2(we)
  Delay46/1 -> data_adc/3(trig)
  Dely47/1 -> oflow_adc/2(we)
  Dely1/1 -> oflow_adc/3(trig)
  Mux1/1 -> oflow_adc/1(din)
  Delay1/1 -> Reinterpret17/1
  Delay3/1 -> Reinterpret18/1
  Delay20/1 -> Reinterpret19/1
  Delay5/1 -> Reinterpret20/1
  Delay4/1 -> Reinterpret21/1
  Delay24/1 -> Reinterpret22/1
  Delay23/1 -> Reinterpret23/1
  Delay26/1 -> Reinterpret24/1
  Delay25/1 -> Reinterpret25/1
  Delay11/1 -> Reinterpret26/1
  Delay10/1 -> Reinterpret27/1
  Delay15/1 -> Reinterpret28/1
  Delay14/1 -> Reinterpret29/1
  Delay13/1 -> Reinterpret30/1
  Delay12/1 -> Reinterpret31/1
  Delay16/1 -> Reinterpret/1
  Reinterpret/1 -> Concat/1
  Reinterpret17/1 -> Concat/2
  Reinterpret18/1 -> Concat/3
  Reinterpret19/1 -> Concat/4
  Reinterpret20/1 -> Concat5/1
  Reinterpret21/1 -> Concat5/2
  Reinterpret22/1 -> Concat5/3
  Reinterpret23/1 -> Concat5/4
  Reinterpret24/1 -> Concat6/1
  Reinterpret25/1 -> Concat6/2
  Reinterpret26/1 -> Concat6/3
  Reinterpret27/1 -> Concat6/4
  Reinterpret28/1 -> Concat7/1
  Reinterpret29/1 -> Concat7/2
  Reinterpret30/1 -> Concat7/3
  Reinterpret31/1 -> Concat7/4
  Concat/1 -> Delay90/1
  ip_select/1 -> Delay89/1
  Concat5/1 -> Delay91/1
  Concat6/1 -> Delay94/1
  Concat7/1 -> Delay96/1
  Mux2/1 -> Slice2/1, Slice1/1, Slice/1, Slice3/1, [adc0_ch0]
  Mux3/1 -> Slice7/1, Slice4/1, Slice5/1, Slice6/1, [adc0_ch1]
  Mux4/1 -> Slice11/1, Slice8/1, Slice9/1, Slice10/1, [adc1_ch0]
  Mux5/1 -> Slice14/1, Slice13/1, Slice12/1, Slice15/1, [adc1_ch1]
  Slice/1 -> Reinterpret48/1
  Slice2/1 -> Reinterpret50/1
  Slice1/1 -> Reinterpret51/1
  Slice3/1 -> Reinterpret49/1
  katadc0/5(or0) -> Delay104/1
  Slice4/1 -> Reinterpret52/1
  Slice7/1 -> Reinterpret53/1
  Slice6/1 -> Reinterpret54/1
  Slice5/1 -> Reinterpret55/1
  katadc1/5(or0) -> Delay107/1
  Slice8/1 -> Reinterpret56/1
  Slice11/1 -> Reinterpret57/1
  Slice10/1 -> Reinterpret58/1
  Slice9/1 -> Reinterpret59/1
  Slice12/1 -> Reinterpret60/1
  Slice15/1 -> Reinterpret61/1
  Slice14/1 -> Reinterpret62/1
  Slice13/1 -> Reinterpret63/1
  Delay83/1 -> Delay122/1
  katadc0/10(or1) -> Delay69/1
  Delay86/1 -> Logical2/1, [adc1_ch0_of]
  katadc1/10(or1) -> Delay80/1
  Delay87/1 -> Logical2/2, [adc1_ch1_of]
  Delay88/1 -> Delay123/1
  Reinterpret48/1 -> Delay72/1
  Reinterpret49/1 -> Delay81/1
  Reinterpret50/1 -> Delay82/1
  Reinterpret51/1 -> Delay109/1
  Reinterpret52/1 -> Delay110/1
  Reinterpret53/1 -> Delay111/1
  Reinterpret54/1 -> Delay112/1
  Reinterpret55/1 -> Delay113/1
  Reinterpret56/1 -> Delay114/1
  Reinterpret57/1 -> Delay115/1
  Reinterpret58/1 -> Delay116/1
  Reinterpret59/1 -> Delay117/1
  Reinterpret60/1 -> Delay118/1
  Reinterpret61/1 -> Delay119/1
  Reinterpret62/1 -> Delay120/1
  Reinterpret63/1 -> Delay121/1
  Delay89/1 -> Slice17/1, Slice16/1, Slice18/1, Slice19/1
  Delay90/1 -> Mux2/2
  Delay91/1 -> Mux3/2
  Delay92/1 -> Delay85/1
  Delay93/1 -> Delay83/1
  Delay94/1 -> Mux4/2
  Delay95/1 -> Delay86/1
  Delay96/1 -> Mux5/2
  Delay97/1 -> Delay87/1
  Delay98/1 -> Delay88/1
  Delay103/1 -> Delay84/1
  Delay104/1 -> Delay105/1
  Delay105/1 -> Delay92/1
  Delay69/1 -> Delay70/1
  Delay70/1 -> Delay103/1
  Delay35/1 -> Delay33/1
  Delay79/1 -> Delay34/1
  Delay80/1 -> Delay106/1
  Delay106/1 -> Delay97/1
  Delay107/1 -> Delay108/1
  Delay108/1 -> Delay95/1
  Logical1/1 -> Delay71/1
  Delay71/1 -> adc0_oflow/1
  Delay72/1 -> adc0_0_0/1
  Delay114/1 -> adc1_0_0/1
  Delay118/1 -> adc1_1_0/1
  Delay85/1 -> Logical1/1, [adc0_ch0_of]
  Delay84/1 -> Logical1/2, [adc0_ch1_of]
  Delay110/1 -> adc0_1_0/1
  Delay81/1 -> adc0_0_1/1
  Delay82/1 -> adc0_0_2/1
  Delay109/1 -> adc0_0_3/1
  Delay111/1 -> adc0_1_1/1
  Delay112/1 -> adc0_1_2/1
  Delay113/1 -> adc0_1_3/1
  Delay119/1 -> adc1_1_1/1
  Delay120/1 -> adc1_1_2/1
  Delay121/1 -> adc1_1_3/1
  Delay117/1 -> adc1_0_3/1
  Delay116/1 -> adc1_0_2/1
  Delay115/1 -> adc1_0_1/1
  Delay122/1 -> adc0_sync/1
  Delay123/1 -> adc1_sync/1
  rst/1 -> Terminator2/1
  Slice17/1 -> Mux2/1
  Slice16/1 -> Mux3/1
  Slice18/1 -> Mux4/1
  Slice19/1 -> Mux5/1
  Constant3/1 -> Mux5/3
  Constant4/1 -> Mux4/3
  Constant5/1 -> Mux3/3
  Constant6/1 -> Mux2/3

== system eovsa_corr_300mhz/adc_overflow ==
  out_reg : Inport
  assert_reg : xbsIndex_r4/Assert  assert_type=on  type_source=Explicitly  gui_display_data_type=Fixed-point  arith_type=Unsigned  n_bits=32  bin_pt=0  preci_type=Single  exp_width=8  frac_width=24  assert_rate=off  rate_source=Explicitly  period=1  output_port=on  block_type=assert
  cast_gw : xbsIndex_r4/Convert  gui_display_data_type=Fixed-point  arith_type=Unsigned  n_bits=32  bin_pt=0  float_type=Single  exp_bits=8  fraction_bits=24  quantization=Truncate  overflow=Wrap  en=off  latency=0  dbl_ovrd=off  pipeline=off  block_type=convert
  eovsa_corr_300mhz_adc_overflow_user_data_in : xbsIndex_r4/Gateway Out  inherit_from_input=off  hdl_port=on  timing_constraint=None  locs_specified=off  LOCs={}  UseAsDAC=off  DACChannel='1'  block_type=gatewayout
  io_delay : xbsIndex_r4/Delay  rst=off  infoeditControl=Selection of Reset will increase slice count due to use of real FFs and instead of SRLs  en=off  latency=0  dbl_ovrd=off  reg_retiming=on  block_type=delay
  reint1 : xbsIndex_r4/Reinterpret  force_arith_type=on  arith_type=Unsigned  force_bin_pt=on  bin_pt=0  block_type=reinterpret
  sim_out : Outport
  wires:
  io_delay/1 -> cast_gw/1
  cast_gw/1 -> eovsa_corr_300mhz_adc_overflow_user_data_in/1
  eovsa_corr_300mhz_adc_overflow_user_data_in/1 -> sim_out/1
  out_reg/1 -> assert_reg/1
  assert_reg/1 -> reint1/1
  reint1/1 -> io_delay/1

== system eovsa_corr_300mhz/armer ==
  target_mcnt : Inport
  vld : Inport  Port=2
  mcnt : Inport  Port=3
  sync : Inport  Port=4
  rst : Inport  Port=5
  data : Inport  Port=6
  Delay{1..12,33} (13 alike) : xbsIndex_r4/Delay  rst=off  infoeditControl=Selection of Reset will increase slice count due to use of real FFs and instead of SRLs  en=off  latency=1  dbl_ovrd=off  reg_retiming=on  block_type=delay
  Logical1 : xbsIndex_r4/Logical  logical_function=AND  inputs=2  en=off  latency=0  precision=Full  arith_type=Unsigned  n_bits=16  bin_pt=0  align_bp=on  dbl_ovrd=off  block_type=logical
  Register4 : xbsIndex_r4/Register  init=0  rst=on  en=on  dbl_ovrd=off  block_type=register
  Register5 : xbsIndex_r4/Register  init=0  rst=off  en=on  dbl_ovrd=off  block_type=register
  Relational : xbsIndex_r4/Relational  mode=a=b  en=off  latency=1  dbl_ovrd=off  block_type=relational
  Slice18 : xbsIndex_r4/Slice  nbits=32  boolean_output=off  mode=Upper Bit Location + Width  bit1=0  base1=MSB of Input  bit0=n_chan_bits  base0=LSB of Input  dbl_ovrd=off  block_type=slice
      settings: block_version=10.1.3
  edge_detect2 : Subsystem  AncestorBlock=casper_library_misc/edge_detect  mask(edge_detect){edge=Rising, polarity=Active High, x_in=[0 0.08 0.08 0.16 0.16 0.24 0.24 0.32 0.32 0.4], y_in=[-1 -1  1  1  1  1  1  1  1  1], x_out=[0.6 0.68 0.68 0.76 0.76 0.84 0.84 0.92 0.92 1], y_out=[-1 -1  1  1 -1 -1 -1 -1 -1 -1]}
      mask prompts: edge "Edge Type"; polarity "Output Polarity"; x_in "Input X Positions"; y_in "Input Y Positions"; x_out "Output X Positions"; y_out "Output Y Positions"
      mask help: Output is active for one-cycle after each edge of the specified type (i.e. rising, falling or both).
      mask init: same as eovsa_corr_300mhz/edge_detect1
      settings: AttributesFormatString=|
      | rising edges
      | active high
      mask Help: Output is active for one-cycle after each edge of the specified type (i.e. rising, falling, or both).  Latency is zero.
      mask TypeOptions edge: Rising | Falling | Both
      mask TypeOptions polarity: Active High | Active Low
      mask Display:
      | plot(x_in_num,0.5+y_in_num*0.2);
      | plot(x_out_num,0.5+y_out_num*0.2);
  sync_out : Outport
  data_out : Outport  Port=2
  vld_out : Outport  Port=3
  mcnt_out : Outport  Port=4
  wires:
  vld/1 -> Delay7/1
  Slice18/1 -> Register5/1
  Register5/1 -> Relational/2
  edge_detect2/1(out) -> Register4/3, Register4/1
  sync/1 -> Delay4/1, Delay33/1
  mcnt/1 -> Delay1/1, Slice18/1
  Delay33/1 -> Register5/2
  target_mcnt/1 -> Relational/1
  Register4/1 -> Logical1/1
  Logical1/1 -> vld_out/1
  Relational/1 -> edge_detect2/1(in)
  Delay1/1 -> Delay2/1
  Delay2/1 -> Delay3/1
  Delay3/1 -> mcnt_out/1
  Delay4/1 -> Delay5/1
  Delay5/1 -> Delay6/1
  Delay6/1 -> sync_out/1
  Delay7/1 -> Delay8/1
  Delay8/1 -> Delay9/1
  Delay9/1 -> Logical1/2
  rst/1 -> Register4/2
  data/1 -> Delay10/1
  Delay10/1 -> Delay11/1
  Delay11/1 -> Delay12/1
  Delay12/1 -> data_out/1

== system eovsa_corr_300mhz/auto_shutoff0 ==
  In1 : Inport
  In2 : Inport  Port=2
  In3 : Inport  Port=3
  In4 : Inport  Port=4
  rst : Inport  Port=5
  Accumulator : xbsIndex_r4/Accumulator  operation=Add  n_bits=ceil(log2(clk_freq*1000*acc_time))+bits_in*2  overflow=Wrap  scale=1  rst=on  infoeditControl=reset for floating point data type must be asserted for a minimum of 2 cycles  hasbypass=off  en=off  latency=0  dbl_ovrd=off  msb_inp=100  msb=100  lsb=-100  use_behavioral_HDL=off  implementation=DSP48  block_type=accum
      settings: xl_area=[0, 0, 0, 0, 0, 0, 0]  block_version=10.1.3
  Constant : xbsIndex_r4/Constant  const=2^ceil(log2(clk_freq*1000*acc_time))*max_power  gui_display_data_type=Fixed-point  arith_type=Unsigned  n_bits=ceil(log2(clk_freq*1000*acc_time))+bits_in*2  bin_pt=bin_pt_in*2  preci_type=Single  exp_width=8  frac_width=24  explicit_period=on  period=1  equ=P=C  opselect=C  inp2=PCIN>>17  opr=+  inp1=P  carry=CIN  dbl_ovrd=off  block_type=constant
      settings: block_version=11.4
  Counter1 : xbsIndex_r4/Counter  cnt_type=Free Running  cnt_to=Inf  operation=Up  start_count=0  cnt_by_val=1  arith_type=Unsigned  n_bits=ceil(log2(clk_freq*1000*acc_time))+1  bin_pt=0  load_pin=off  rst=off  en=off  explicit_period=on  period=1  dbl_ovrd=off  use_behavioral_HDL=off  implementation=DSP48  use_rpm=on  block_type=counter
      settings: xl_area=[0, 0, 0, 0, 0, 0, 0]
  Counter2 : xbsIndex_r4/Counter  cnt_type=Free Running  cnt_to=Inf  operation=Up  start_count=0  cnt_by_val=1  arith_type=Unsigned  n_bits=2  bin_pt=0  load_pin=off  rst=off  en=off  explicit_period=on  period=1  dbl_ovrd=off  use_behavioral_HDL=off  implementation=Fabric  block_type=counter
      settings: block_version=11.4
  Delay4 : xbsIndex_r4/Delay  rst=off  infoeditControl=Selection of Reset will increase slice count due to use of real FFs and instead of SRLs  en=off  latency=1  dbl_ovrd=off  reg_retiming=off  block_type=delay
      settings: block_version=11.4
  Logical : xbsIndex_r4/Logical  logical_function=OR  inputs=2  en=off  latency=1  precision=Full  arith_type=Unsigned  n_bits=16  bin_pt=0  align_bp=on  dbl_ovrd=off  block_type=logical
      settings: block_version=11.4
  Mult : xbsIndex_r4/Mult  precision=Full  arith_type="Signed  (2's comp)"  n_bits=8  bin_pt=2  quantization=Truncate  overflow=Wrap  en=off  latency=3  dbl_ovrd=off  use_behavioral_HDL=off  opt=Speed  use_embedded=on  optimum_pipeline=off  pipeline=on  use_rpm=on  placement_style=Rectangular shape  block_type=mult
      settings: xl_area=[0, 0, 0, 0, 0, 0, 0]  block_version=10.1.3
  Mux : xbsIndex_r4/Mux  inputs=4  en=off  latency=1  precision=Full  arith_type="Signed  (2's comp)"  n_bits=8  bin_pt=2  quantization=Truncate  overflow=Wrap  dbl_ovrd=off  block_type=mux
      settings: xl_area=[0, 0, 0, 0, 0, 0, 0]
  Relational : xbsIndex_r4/Relational  mode=a>b  en=off  latency=1  dbl_ovrd=off  block_type=relational
  Slice : xbsIndex_r4/Slice  nbits=1  boolean_output=off  mode=Upper Bit Location + Width  bit1=0  base1=MSB of Input  bit0=0  base0=LSB of Input  dbl_ovrd=off  block_type=slice
      settings: block_version=10.1.3
  Slice1 : xbsIndex_r4/Slice  nbits=1  boolean_output=on  mode=Upper Bit Location + Width  bit1=0  base1=MSB of Input  bit0=0  base0=LSB of Input  dbl_ovrd=off  block_type=slice
  edge_detect : Subsystem  AncestorBlock=casper_library_misc/edge_detect  mask(edge_detect){edge=Both, polarity=Active High, x_in=[0 0.08 0.08 0.16 0.16 0.24 0.24 0.32 0.32 0.4], y_in=[-1 -1  1  1  1  1 -1 -1 -1 -1], x_out=[0.6 0.68 0.68 0.76 0.76 0.84 0.84 0.92 0.92 1], y_out=[-1 -1  1  1 -1 -1  1  1 -1 -1]}
      mask prompts: edge "Edge Type"; polarity "Output Polarity"; x_in "Input X Positions"; y_in "Input Y Positions"; x_out "Output X Positions"; y_out "Output Y Positions"
      mask help: Output is active for one-cycle after each edge of the specified type (i.e. rising, falling or both).
      mask init: same as eovsa_corr_300mhz/edge_detect1
      settings: AttributesFormatString=|
      | both edges
      | active high
      mask Help: Output is active for one-cycle after each edge of the specified type (i.e. rising, falling, or both).  Latency is zero.
      mask TypeOptions edge: Rising | Falling | Both
      mask TypeOptions polarity: Active High | Active Low
      mask Display:
      | plot(x_in_num,0.5+y_in_num*0.2);
      | plot(x_out_num,0.5+y_out_num*0.2);
  en : Outport
  wires:
  Slice1/1 -> Logical/1
  Mult/1 -> Delay4/1
  Accumulator/1 -> Relational/1
  Counter1/1 -> Slice/1
  Slice/1 -> edge_detect/1(in)
  Mux/1 -> Mult/1, Mult/2
  Counter2/1 -> Mux/1
  In1/1 -> Mux/2
  In3/1 -> Mux/3
  In2/1 -> Mux/4
  In4/1 -> Mux/5
  Constant/1 -> Relational/2
  Relational/1 -> en/1
  rst/1 -> Logical/2
  edge_detect/1(out) -> Slice1/1
  Logical/1 -> Accumulator/2
  Delay4/1 -> Accumulator/1
